simulink model "CTC_2LinkManipulator"  (R2022b)
settings: Solver=FixedStepAuto  StartTime=0.0  StopTime=10  FixedStep=0.001  RelTol=1e-3
values from neighbouring files (symbols this model uses):
  dynSwitch = 0    [twoLink_Init.m]
  Kd = [40,0;0,80]    [twoLink_Init.m]
  Kp = [11,0;0,18]    [twoLink_Init.m]
  q1_dot_init = 0    [twoLink_Init.m]
  q1_init = 0.5    [twoLink_Init.m]
  q2_dot_init = 0    [twoLink_Init.m]
  q2_init = 0.5    [twoLink_Init.m]
  simActual = struct()    [twoLink_Init.m]
  simNominal = struct()    [twoLink_Init.m]
settings Model: Creator=ashut  LastModifiedBy=ashut

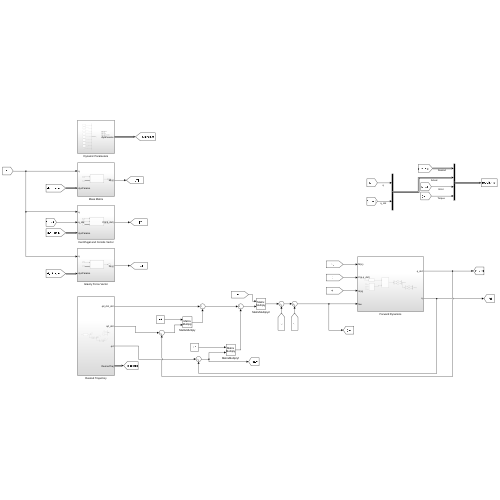
[thumbnail: Simulink's stored preview of the top-level diagram]
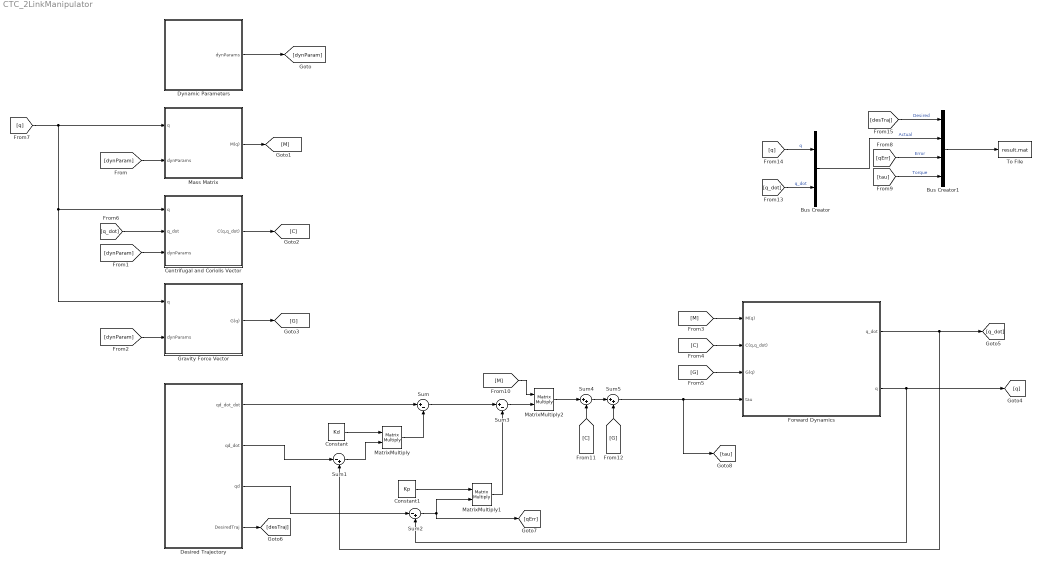
== system CTC_2LinkManipulator ==
  Bus Creator : BusCreator  Inputs=2
  Bus Creator1 : BusCreator  Inputs=4
  Centrifugal and Coriolis Vector : Subsystem
  Constant : Constant  Value=Kd
  Constant1 : Constant  Value=Kp
  Desired Trajectory : Subsystem
  Dynamic Parameters : Subsystem
  Forward Dynamics : Subsystem
  Gravity Force Vector : Subsystem
  Mass Matrix : Subsystem
  MatrixMultiply : Product  Multiplication=Matrix(*)
  MatrixMultiply1 : Product  Multiplication=Matrix(*)
  MatrixMultiply2 : Product  Multiplication=Matrix(*)
  Sum : Sum  Inputs=|+-
  Sum1 : Sum  Inputs=|-+
  Sum2 : Sum  Inputs=|-+
  Sum3 : Sum  Inputs=|+-
  Sum4 : Sum  Inputs=|++
  Sum5 : Sum  Inputs=|++
  To File : ToFile  Filename=result.mat  SaveFormat=Timeseries
  wires:
  Dynamic Parameters/1(dynParams) -> [dynParam]
  [dynParam] -> Mass Matrix/2(dynParams)
  [dynParam] -> Centrifugal and Coriolis Vector/3(dynParams)
  [dynParam] -> Gravity Force Vector/2(dynParams)
  Mass Matrix/1(M(q)) -> [M]
  Centrifugal and Coriolis Vector/1(C(q,q_dot)) -> [C]
  Gravity Force Vector/1(G(q)) -> [G]
  [M] -> Forward Dynamics/1(M(q))
  [C] -> Forward Dynamics/2(C(q,q_dot))
  [G] -> Forward Dynamics/3(G(q))
  Forward Dynamics/2(q) -> Sum2/2, [q]
  Forward Dynamics/1(q_dot) -> Sum1/2, [q_dot]
  Desired Trajectory/2(qd_dot) -> Sum1/1
  Constant/1 -> MatrixMultiply/1
  Sum1/1 -> MatrixMultiply/2
  MatrixMultiply/1 -> Sum/2
  Constant1/1 -> MatrixMultiply1/1
  Sum2/1 -> [qErr], MatrixMultiply1/2
  Desired Trajectory/1(qd_dot_dot) -> Sum/1
  Desired Trajectory/3(qd) -> Sum2/1
  MatrixMultiply1/1 -> Sum3/2
  Sum/1 -> Sum3/1
  [M] -> MatrixMultiply2/1
  Sum3/1 -> MatrixMultiply2/2
  MatrixMultiply2/1 -> Sum4/1
  [C] -> Sum4/2
  Sum4/1 -> Sum5/1
  [G] -> Sum5/2
  Sum5/1 -> [tau], Forward Dynamics/4(tau)
  Desired Trajectory/4(DesiredTraj) -> [desTraj]
  [q] -> Bus Creator/1  "q"
  [q_dot] -> Bus Creator/2  "q_dot"
  [desTraj] -> Bus Creator1/1  "Desired"
  Bus Creator/1 -> Bus Creator1/2  "Actual"
  Bus Creator1/1 -> To File/1
  [q] -> Gravity Force Vector/1(q), Centrifugal and Coriolis Vector/1(q), Mass Matrix/1(q)
  [q_dot] -> Centrifugal and Coriolis Vector/2(q_dot)
  [qErr] -> Bus Creator1/3  "Error"
  [tau] -> Bus Creator1/4  "Torque"

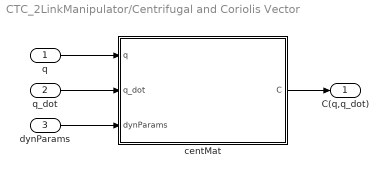
== system CTC_2LinkManipulator/Centrifugal and Coriolis Vector ==
  q : Inport
  q_dot : Inport  Port=2
  dynParams : Inport  Port=3
  centMat : MATLAB Function  TreatAsAtomicUnit=on
  C(q,q_dot) : Outport
  wires:
  centMat/1(C) -> C(q,q_dot)/1
  dynParams/1 -> centMat/3(dynParams)
  q/1 -> centMat/1(q)
  q_dot/1 -> centMat/2(q_dot)

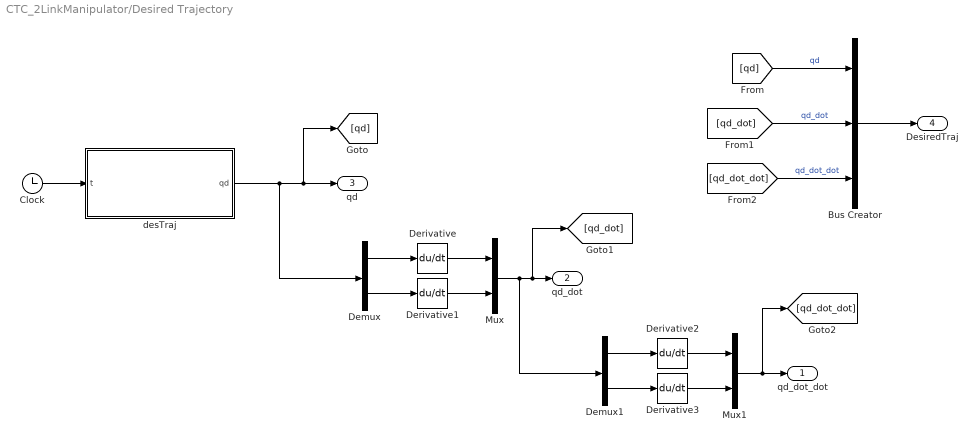
== system CTC_2LinkManipulator/Desired Trajectory ==
  Bus Creator : BusCreator  Inputs=3
  Clock : Clock
  Demux : Demux  Outputs=2
  Demux1 : Demux  Outputs=2
  Derivative{,1..3} (4 alike) : Derivative
  Mux : Mux  Inputs=2
  Mux1 : Mux  Inputs=2
  desTraj : MATLAB Function  TreatAsAtomicUnit=on
  qd_dot_dot : Outport
  qd_dot : Outport  Port=2
  qd : Outport  Port=3
  DesiredTraj : Outport  Port=4
  wires:
  Clock/1 -> desTraj/1(t)
  desTraj/1(qd) -> Demux/1, [qd], qd/1
  Derivative1/1 -> Mux/2
  Derivative/1 -> Mux/1
  Demux/1 -> Derivative/1
  Demux/2 -> Derivative1/1
  Mux1/1 -> [qd_dot_dot], qd_dot_dot/1
  Demux1/2 -> Derivative3/1
  Demux1/1 -> Derivative2/1
  Derivative2/1 -> Mux1/1
  Derivative3/1 -> Mux1/2
  Mux/1 -> Demux1/1, [qd_dot], qd_dot/1
  [qd_dot] -> Bus Creator/2  "qd_dot"
  [qd_dot_dot] -> Bus Creator/3  "qd_dot_dot"
  [qd] -> Bus Creator/1  "qd"
  Bus Creator/1 -> DesiredTraj/1

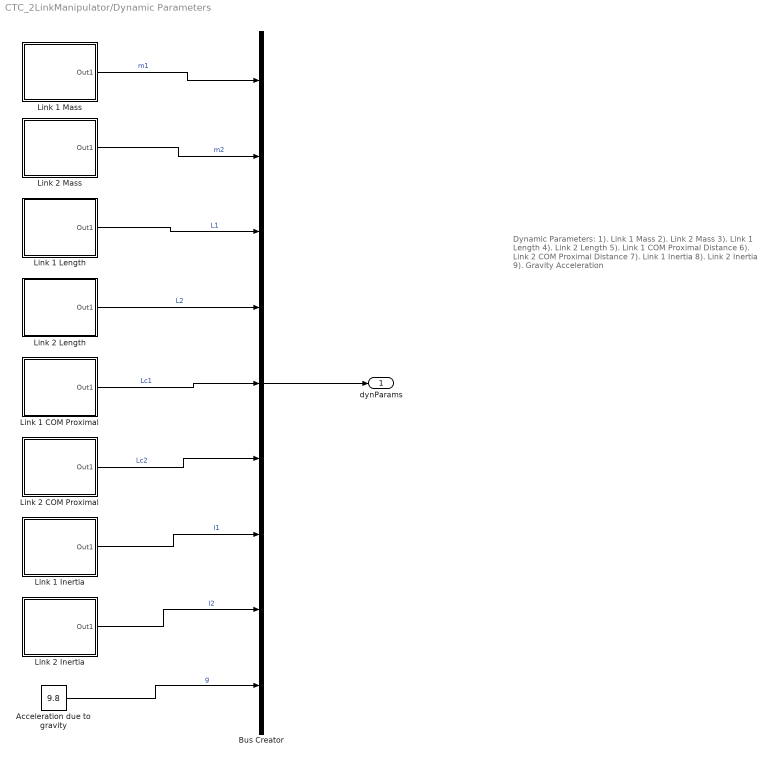
== system CTC_2LinkManipulator/Dynamic Parameters ==
  note: Dynamic Parameters:
      | 1). Link 1 Mass
      | 2). Link 2 Mass
      | 3). Link 1 Length
      | 4). Link 2 Length
      | 5). Link 1 COM Proximal Distance
      | 6). Link 2 COM Proximal Distance
      | 7). Link 1 Inertia
      | 8). Link 2 Inertia
      | 9). Gravity Acceleration
  Acceleration due to gravity : Constant  Value=9.8
  Bus Creator : BusCreator  Inputs=9
  Link 1 COM Proximal : Subsystem
  Link 1 Inertia : Subsystem
  Link 1 Length : Subsystem
  Link 1 Mass : Subsystem
  Link 2 COM Proximal : Subsystem
  Link 2 Inertia : Subsystem
  Link 2 Length : Subsystem
  Link 2 Mass : Subsystem
  dynParams : Outport
  wires:
  Link 2 Length/1(Out1) -> Bus Creator/4  "L2"
  Link 1 Mass/1(Out1) -> Bus Creator/1  "m1"
  Link 2 COM Proximal/1(Out1) -> Bus Creator/6  "Lc2"
  Link 1 Inertia/1(Out1) -> Bus Creator/7  "I1"
  Link 2 Inertia/1(Out1) -> Bus Creator/8  "I2"
  Link 2 Mass/1(Out1) -> Bus Creator/2  "m2"
  Bus Creator/1 -> dynParams/1
  Link 1 Length/1(Out1) -> Bus Creator/3  "L1"
  Link 1 COM Proximal/1(Out1) -> Bus Creator/5  "Lc1"
  Acceleration due to gravity/1 -> Bus Creator/9  "g"

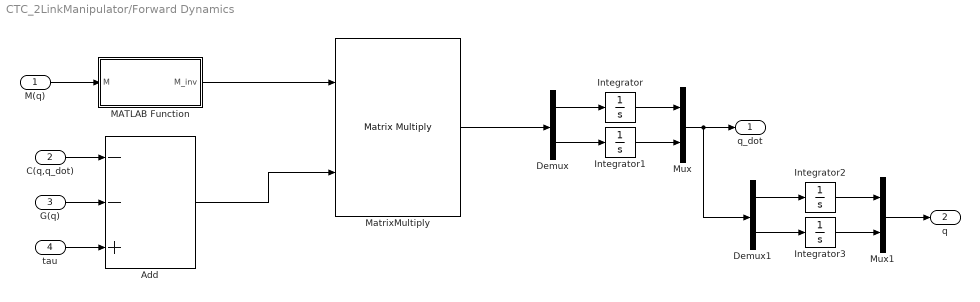
== system CTC_2LinkManipulator/Forward Dynamics ==
  M(q) : Inport
  C(q,q_dot) : Inport  Port=2
  G(q) : Inport  Port=3
  tau : Inport  Port=4
  Add : Sum  Inputs=--+
  Demux : Demux  Outputs=2
  Demux1 : Demux  Outputs=2
  Integrator : Integrator  InitialCondition=q1_dot_init
  Integrator1 : Integrator  InitialCondition=q2_dot_init
  Integrator2 : Integrator  InitialCondition=q1_init
  Integrator3 : Integrator  InitialCondition=q2_init
  MATLAB Function : MATLAB Function  TreatAsAtomicUnit=on
  MatrixMultiply : Product  Multiplication=Matrix(*)
  Mux : Mux  Inputs=2
  Mux1 : Mux  Inputs=2
  q_dot : Outport  PortDimensions=2
  q : Outport  Port=2  PortDimensions=2
  wires:
  M(q)/1 -> MATLAB Function/1(M)
  MATLAB Function/1(M_inv) -> MatrixMultiply/1
  Add/1 -> MatrixMultiply/2
  MatrixMultiply/1 -> Demux/1
  Demux/1 -> Integrator/1
  Demux/2 -> Integrator1/1
  Integrator1/1 -> Mux/2
  Integrator/1 -> Mux/1
  Mux1/1 -> q/1
  Integrator2/1 -> Mux1/1
  Integrator3/1 -> Mux1/2
  Demux1/2 -> Integrator3/1
  Demux1/1 -> Integrator2/1
  Mux/1 -> Demux1/1, q_dot/1
  G(q)/1 -> Add/2
  C(q,q_dot)/1 -> Add/1
  tau/1 -> Add/3

== system CTC_2LinkManipulator/Gravity Force Vector ==
  q : Inport
  dynParams : Inport  Port=2
  gravMat : MATLAB Function  TreatAsAtomicUnit=on
  G(q) : Outport
  wires:
  gravMat/1(G) -> G(q)/1
  dynParams/1 -> gravMat/2(dynParams)
  q/1 -> gravMat/1(q)

== system CTC_2LinkManipulator/Mass Matrix ==
  q : Inport
  dynParams : Inport  Port=2
  massMat : MATLAB Function  TreatAsAtomicUnit=on
  M(q) : Outport
  wires:
  q/1 -> massMat/1(q)
  dynParams/1 -> massMat/2(dynParams)
  massMat/1(M) -> M(q)/1

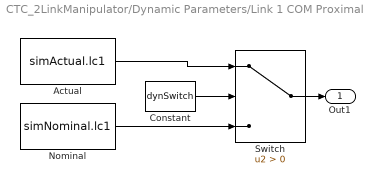
== system CTC_2LinkManipulator/Dynamic Parameters/Link 1 COM Proximal ==
  "Actual " : Constant  Value=simActual.lc1
  Constant : Constant  Value=dynSwitch
  Nominal : Constant  Value=simNominal.lc1
  Switch : Switch  Criteria=u2 > Threshold  SaturateOnIntegerOverflow=off  InputSameDT=off
  Out1 : Outport
  wires:
  Switch/1 -> Out1/1
  Nominal/1 -> Switch/3
  "Actual "/1 -> Switch/1
  Constant/1 -> Switch/2

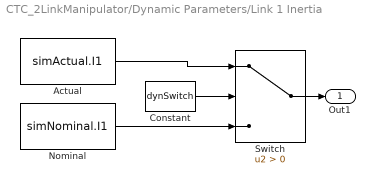
== system CTC_2LinkManipulator/Dynamic Parameters/Link 1 Inertia ==
  "Actual " : Constant  Value=simActual.I1
  Constant : Constant  Value=dynSwitch
  Nominal : Constant  Value=simNominal.I1
  Switch : Switch  Criteria=u2 > Threshold  SaturateOnIntegerOverflow=off  InputSameDT=off
  Out1 : Outport
  wires:
  Constant/1 -> Switch/2
  "Actual "/1 -> Switch/1
  Nominal/1 -> Switch/3
  Switch/1 -> Out1/1

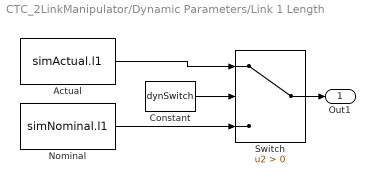
== system CTC_2LinkManipulator/Dynamic Parameters/Link 1 Length ==
  "Actual " : Constant  Value=simActual.l1
  Constant : Constant  Value=dynSwitch
  Nominal : Constant  Value=simNominal.l1
  Switch : Switch  Criteria=u2 > Threshold  SaturateOnIntegerOverflow=off  InputSameDT=off
  Out1 : Outport
  wires:
  Constant/1 -> Switch/2
  "Actual "/1 -> Switch/1
  Nominal/1 -> Switch/3
  Switch/1 -> Out1/1

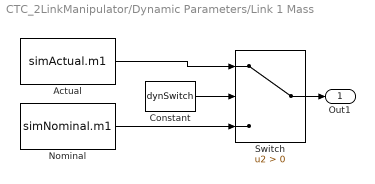
== system CTC_2LinkManipulator/Dynamic Parameters/Link 1 Mass ==
  "Actual " : Constant  Value=simActual.m1
  Constant : Constant  Value=dynSwitch
  Nominal : Constant  Value=simNominal.m1
  Switch : Switch  Criteria=u2 > Threshold  SaturateOnIntegerOverflow=off  InputSameDT=off
  Out1 : Outport
  wires:
  Constant/1 -> Switch/2
  "Actual "/1 -> Switch/1
  Nominal/1 -> Switch/3
  Switch/1 -> Out1/1

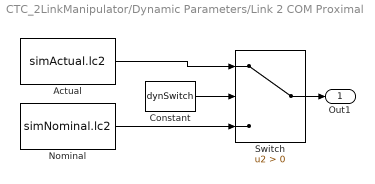
== system CTC_2LinkManipulator/Dynamic Parameters/Link 2 COM Proximal ==
  "Actual " : Constant  Value=simActual.lc2
  Constant : Constant  Value=dynSwitch
  Nominal : Constant  Value=simNominal.lc2
  Switch : Switch  Criteria=u2 > Threshold  SaturateOnIntegerOverflow=off  InputSameDT=off
  Out1 : Outport
  wires:
  Constant/1 -> Switch/2
  "Actual "/1 -> Switch/1
  Nominal/1 -> Switch/3
  Switch/1 -> Out1/1

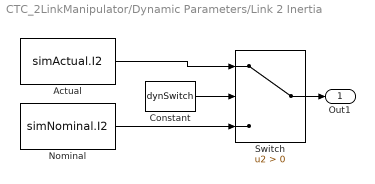
== system CTC_2LinkManipulator/Dynamic Parameters/Link 2 Inertia ==
  "Actual " : Constant  Value=simActual.I2
  Constant : Constant  Value=dynSwitch
  Nominal : Constant  Value=simNominal.I2
  Switch : Switch  Criteria=u2 > Threshold  SaturateOnIntegerOverflow=off  InputSameDT=off
  Out1 : Outport
  wires:
  Switch/1 -> Out1/1
  Nominal/1 -> Switch/3
  "Actual "/1 -> Switch/1
  Constant/1 -> Switch/2

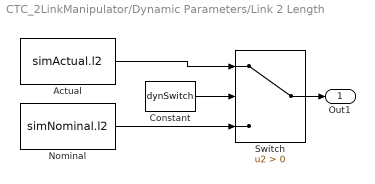
== system CTC_2LinkManipulator/Dynamic Parameters/Link 2 Length ==
  "Actual " : Constant  Value=simActual.l2
  Constant : Constant  Value=dynSwitch
  Nominal : Constant  Value=simNominal.l2
  Switch : Switch  Criteria=u2 > Threshold  SaturateOnIntegerOverflow=off  InputSameDT=off
  Out1 : Outport
  wires:
  Switch/1 -> Out1/1
  Nominal/1 -> Switch/3
  "Actual "/1 -> Switch/1
  Constant/1 -> Switch/2

== system CTC_2LinkManipulator/Dynamic Parameters/Link 2 Mass ==
  "Actual " : Constant  Value=simActual.m2
  Constant : Constant  Value=dynSwitch
  Nominal : Constant  Value=simNominal.m2
  Switch : Switch  Criteria=u2 > Threshold  SaturateOnIntegerOverflow=off  InputSameDT=off
  Out1 : Outport
  wires:
  Switch/1 -> Out1/1
  Nominal/1 -> Switch/3
  "Actual "/1 -> Switch/1
  Constant/1 -> Switch/2

== matlab function CTC_2LinkManipulator/Mass Matrix/massMat ==
  data: q input; M output; dynParams input
function M = massMat(q,dynParams)
m1 = dynParams(1);
m2 = dynParams(2);
l1 = dynParams(3);
l2 = dynParams(4);
lc1 = dynParams(5);
lc2 = dynParams(6);
I1 = dynParams(7);
I2 = dynParams(8);
m11 = m1*lc1*lc1 + m2*(l1*l1 + lc2*lc2) + 2*m2*l1*lc2*cos(q(2)) + I1 + I2;
m12 = m2*lc2*lc2 + m2*l1*lc2*cos(q(2)) + I2;
m21 = m12;
m22 = m2*lc2*lc2 + I2;
M = [m11,m12;
    m21,m22];

== matlab function CTC_2LinkManipulator/Gravity Force Vector/gravMat ==
  data: q input; G output; dynParams input
function G = gravMat(q,dynParams)
m1 = dynParams(1);
m2 = dynParams(2);
l1 = dynParams(3);
l2 = dynParams(4);
lc1 = dynParams(5);
lc2 = dynParams(6);
g = dynParams(9);
g1 = m1*lc1*g*cos(q(1)) + m2*g*(lc2*cos(q(1) + q(2)) + l1*cos(q(1)));
g2 = m2*lc2*g*cos(q(1) + q(2));
G = [g1;g2];

== matlab function CTC_2LinkManipulator/Desired Trajectory/desTraj ==
  data: t input; qd output
function qd = desTraj(t)

qd1 = (1-exp(-0.05*t))*sin(pi*t);
qd2 = (1-exp(-0.05*t))*sin(pi*t);
qd = [qd1;qd2];

== matlab function CTC_2LinkManipulator/Forward Dynamics/MATLAB Function ==
  data: M input; M_inv output
function M_inv = invertM(M)

M_inv = M\eye(size(M));

== matlab function CTC_2LinkManipulator/Centrifugal and Coriolis Vector/centMat ==
  data: q input; q_dot input; C output; dynParams input
function C = centMat(q,q_dot,dynParams)
m1 = dynParams(1);
m2 = dynParams(2);
l1 = dynParams(3);
l2 = dynParams(4);
lc1 = dynParams(5);
lc2 = dynParams(6);
I1 = dynParams(7);
I2 = dynParams(8);
c1 = -2*m2*l1*lc2*q_dot(1)*q_dot(2)*sin(q(2)) - m2*l1*lc2*q_dot(2)*q_dot(2)*sin(q(2));
c2 = m2*l1*lc2*q_dot(1)*q_dot(1)*sin(q(2));
C = [c1;c2];
